simulink model "rtwdemo_tfladdsub"  (Simulink 7.6)
settings: Solver=ode3  StartTime=0.0  StopTime=20  FixedStep=1  RelTol=1e-3  SampleTimeConstraint=Specified
PreLoadFcn:
  | addpath(fullfile(matlabroot,'toolbox','rtw','rtwdemos','tfl_demo'));
  | sl_refresh_customizations;
libraries: rtwdemowidgets x2
settings Model: Creator=The MathWorks Inc.  ExtModeAutoUpdateStatusClock=off
settings MATStruct: SampleTime=1  Offset=0  Priority=[30.0]
settings DataIOCC: SaveOutput=off  SaveTime=off  SignalLoggingName=sigsOut
settings OptimizationCC: InlineParams=on  InlineInvariantSignals=on  PassReuseOutputArgsAs=Individual arguments  StateBitsets=on  DataBitsets=on  UseTempVars=on  ZeroExternalMemoryAtStartup=off  ZeroInternalMemoryAtStartup=off  NoFixptDivByZeroProtection=on  EfficientFloat2IntCast=on  EfficientMapNaN2IntZero=off  OptimizeModelRefInitCode=on  LifeSpan=1
settings DebuggingCC: CheckExecutionContextPreStartOutputMsg=on  CheckExecutionContextRuntimeOutputMsg=on  SolverPrmCheckMsg=none  StrictBusMsg=ErrorOnBusTreatedAsVector
settings HardwareCC: ProdIntDivRoundTo=Zero  ProdEndianess=LittleEndian  ProdHWDeviceType=Generic->32-bit Embedded Processor  TargetHWDeviceType=32-bit Generic
settings SFSimCC: SimParseCustomCode=off
settings RTWCC: SystemTargetFile=ert.tlc  GenCodeOnly=on  TemplateMakefile=ert_default_tmf  Description=Real-Time Workshop Embedded Coder (no auto configuration)  GenerateReport=on  RTWVerbose=off  ProcessScript=ert_make_rtw_hook  IncludeHyperlinkInReport=on  LaunchReport=on
settings CodeAppCC: ForceParamTrailComments=on  IgnoreCustomStorageClasses=off  IgnoreTestpoints=on  SimulinkDataObjDesc=on  CustomSymbolStrGlobalVar=rt$N$M  CustomSymbolStrType=$N$M  CustomSymbolStrFcn=$N$M$F  CustomSymbolStrMacro=$N$M  InsertBlockDesc=on
settings ERTTargetCC: TargetFunctionLibrary=Addition & Subtraction Examples  MultiwordLength=2048  GenerateSampleERTMain=on  IncludeMdlTerminateFcn=off  SupportNonFinite=off  SupportComplex=off  InlinedParameterPlacement=NonHierarchical  ERTCustomFileTemplate=example_file_process.tlc  ConvertIfToSwitch=off

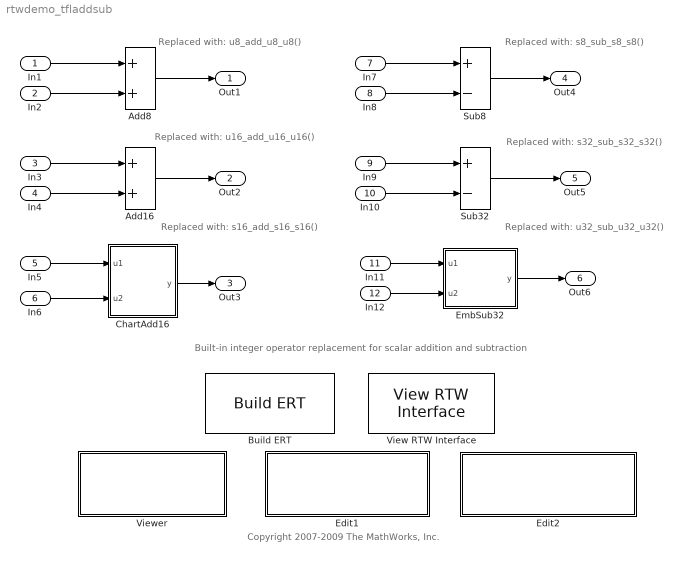
== system rtwdemo_tfladdsub ==
  note: Copyright 2007-2009 The MathWorks, Inc.
  note: Replaced with:
      | u8_add_u8_u8()
  note: Replaced with:
      | s32_sub_s32_s32()
  note: Replaced with:
      | u16_add_u16_u16()
  note: Replaced with:
      | u32_sub_u32_u32()
  note: Built-in integer operator replacement for scalar addition and subtraction
  note: Replaced with:
      | s16_add_s16_s16()
  note: Replaced with:
      | s8_sub_s8_s8()
  In1 : Inport  OutDataTypeStr=uint8  PortDimensions=1  SampleTime=1
  In2 : Inport  Port=2  OutDataTypeStr=uint8  PortDimensions=1  SampleTime=1
  In3 : Inport  Port=3  OutDataTypeStr=uint16  PortDimensions=1  SampleTime=1
  In4 : Inport  Port=4  OutDataTypeStr=uint16  PortDimensions=1  SampleTime=1
  In5 : Inport  Port=5  OutDataTypeStr=int16  PortDimensions=1  SampleTime=1
  In6 : Inport  Port=6  OutDataTypeStr=int16  PortDimensions=1  SampleTime=1
  In7 : Inport  Port=7  OutDataTypeStr=int8  PortDimensions=1  SampleTime=1
  In8 : Inport  Port=8  OutDataTypeStr=int8  PortDimensions=1  SampleTime=1
  In9 : Inport  Port=9  OutDataTypeStr=int32  PortDimensions=1  SampleTime=1
  In10 : Inport  Port=10  OutDataTypeStr=int32  PortDimensions=1  SampleTime=1
  In11 : Inport  Port=11  OutDataTypeStr=uint32  PortDimensions=1  SampleTime=1
  In12 : Inport  Port=12  OutDataTypeStr=uint32  PortDimensions=1  SampleTime=1
  Add16 : Sum  OutDataTypeStr=uint16  RndMeth=Ceiling
  Add8 : Sum  OutDataTypeStr=uint8  SaturateOnIntegerOverflow=on
  Build ERT : rtwdemowidgets/Build ERT  SystemSampleTime=-1  attrib_overrides={'GenFloatMathFcnCalls'}
  ChartAdd16 : Stateflow chart  TreatAsAtomicUnit=on
  Edit1 : Subsystem  mask{attrib_overrides={}}
      mask prompts: attrib_overrides "List of attributes to preserve (cell of strings):"
      mask help: Enter the attributes of the configuration set that you want preserved. Otherwise, the default configuration script will override your current settings.
      settings: OpenFcn=edit('tfl_table_addsub.m');
      mask Display:
      | disp(['View/edit TFL Definition \n',...
      | 	  'tfl_table_addsub.m\n(double-click)'])
  Edit2 : Subsystem  mask{attrib_overrides={}}
      mask prompts: attrib_overrides "List of attributes to preserve (cell of strings):"
      mask help: Enter the attributes of the configuration set that you want preserved. Otherwise, the default configuration script will override your current settings.
      settings: OpenFcn=edit(fullfile(matlabroot,'toolbox','rtw','rtwdemos','tfl_demo', 'sl_customization.m'));
      mask Display:
      | disp(['View/edit TFL Registration \n',...
      | 	  'sl_customization.m\n(double-click)'])
  EmbSub32 : Stateflow chart  TreatAsAtomicUnit=on
  Sub32 : Sum  Inputs=+-  OutDataTypeStr=int32
  Sub8 : Sum  Inputs=+-  OutDataTypeStr=int8  RndMeth=Nearest  SaturateOnIntegerOverflow=on
  View RTW Interface : rtwdemowidgets/View RTW Interface  SystemSampleTime=-1
  Viewer : Subsystem  mask{attrib_overrides={}}
      mask prompts: attrib_overrides "List of attributes to preserve (cell of strings):"
      mask help: Enter the attributes of the configuration set that you want preserved. Otherwise, the default configuration script will override your current settings.
      settings: OpenFcn=|
      | tfl = tfl_table_addsub;
      | obj = RTW.viewTfl(tfl);
      | clear tfl obj;
      mask Display:
      | disp(['Invoke TFL Viewer on\n',...
      | 	  'tfl_table_addsub.m\n(double-click)'])
  Out1 : Outport
  Out2 : Outport  Port=2
  Out3 : Outport  Port=3
  Out4 : Outport  Port=4
  Out5 : Outport  Port=5
  Out6 : Outport  Port=6
  wires:
  Add8/1 -> Out1/1
  In1/1 -> Add8/1
  In2/1 -> Add8/2
  Sub32/1 -> Out5/1
  In9/1 -> Sub32/1
  In3/1 -> Add16/1
  Add16/1 -> Out2/1
  In10/1 -> Sub32/2
  In11/1 -> EmbSub32/1(u1)
  In12/1 -> EmbSub32/2(u2)
  EmbSub32/1(y) -> Out6/1
  In4/1 -> Add16/2
  ChartAdd16/1(y) -> Out3/1
  In6/1 -> ChartAdd16/2(u2)
  In5/1 -> ChartAdd16/1(u1)
  Sub8/1 -> Out4/1
  In7/1 -> Sub8/1
  In8/1 -> Sub8/2

== system rtwdemo_tfladdsub/Edit1 ==

== system rtwdemo_tfladdsub/Edit2 ==

== system rtwdemo_tfladdsub/Viewer ==

== matlab function EmbSub32 ==
  data: u1 input uint32; y output uint32; u2 input uint32
function y = fcn(u1, u2)
% This block supports the Embedded MATLAB subset.
% See the help menu for details. 

assert(isa(u1,'uint32'));
assert(isa(u2,'uint32'));

y = u1-u2;

== stateflow chart ChartAdd16 ==
  (default) -> (junction 11) : {y := u1+u2;}
  data: u1 input int16; u2 input int16; y output int16
